simulink model "untitled2"  (R2016a)
settings: Solver=VariableStepAuto  StartTime=0.0  StopTime=50  RelTol=1e-3
settings Model: Creator=Student  LastModifiedBy=Student

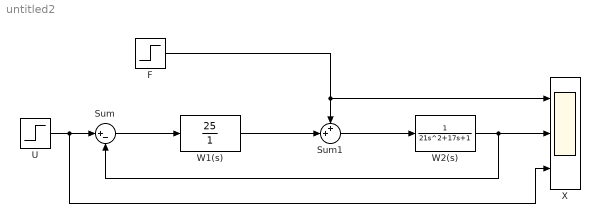
== system untitled2 ==
  F : Step  After=5  SampleTime=0
  Sum : Sum  Inputs=|+-
  Sum1 : Sum  Inputs=++|
  U : Step  SampleTime=0
  W1(s) : TransferFcn  Numerator=[25]  Denominator=[1]
  W2(s) : TransferFcn  Denominator=[21 17 1]
  X : Scope  NumInputPorts=3
  wires:
  U/1 -> X/3, Sum/1
  Sum/1 -> W1(s)/1
  Sum1/1 -> W2(s)/1
  W2(s)/1 -> Sum/2, X/2
  W1(s)/1 -> Sum1/2
  F/1 -> X/1, Sum1/1
